simulink model "EZEStEnCtrl"  (R2018b)
settings: Solver=FixedStepDiscrete  StartTime=0.0  StopTime=10.0  FixedStep=0.01  RelTol=1e-3  EnableMultiTasking=on
undefined symbols (not defined in the file or in its folder): data, DrvStFtEn_Clear, DrvStFtEn_Set, KeSMSwSecRwLtStEasyEntryCllsnPt_Val, KeSMSwSecRwRtStEasyEntryCllsnPt_Val, PassStFtEn_Clear, PassStFtEn_Set, SecRwLtStArmScrnEn_Clear, SecRwLtStArmScrnEn_Set, SecRwLtStBkReclnEn_Clear, SecRwLtStBkReclnEn_Set, SecRwLtStFwdBkwdEn_Clear, SecRwLtStFwdBkwdEn_Set, SecRwLtStLgrstUpwdDnwdEn_Clear, SecRwLtStLgrstUpwdDnwdEn_Set, SecRwLtStLtwdRtwdEn_Clear, SecRwLtStLtwdRtwdEn_Set, SecRwRtStArmScrnEn_Clear, SecRwRtStArmScrnEn_Set, SecRwRtStBkReclnEn_Clear, SecRwRtStBkReclnEn_Set, SecRwRtStFwdBkwdEn_Clear, SecRwRtStFwdBkwdEn_Set, SecRwRtStLgrstUpwdDnwdEn_Clear, SecRwRtStLgrstUpwdDnwdEn_Set, SecRwRtStLtwdRtwdEn_Clear, SecRwRtStLtwdRtwdEn_Set, ThdRwLtStBkReclnEn_Clear, ThdRwLtStBkReclnEn_Set, ThdRwLtStCshnFldEn_Clear, ThdRwLtStCshnFldEn_Set, ThdRwLtStFwdBkwdEn_Clear, ThdRwLtStFwdBkwdEn_Set, ThdRwRtStBkReclnEn_Clear, ThdRwRtStBkReclnEn_Set, ThdRwRtStCshnFldEn_Clear, ThdRwRtStCshnFldEn_Set, ThdRwRtStFwdBkwdEn_Clear, ThdRwRtStFwdBkwdEn_Set
libraries: simulink x1
settings Model: Creator=sn2xws  LastModifiedBy=sn2xws
settings DataIOCC: SaveFormat=StructureWithTime
settings OptimizationCC: DefaultParameterBehavior=Inlined  UseFloatMulNetSlope=on  InlineInvariantSignals=on  PassReuseOutputArgsAs=Individual arguments  ZeroExternalMemoryAtStartup=off  ZeroInternalMemoryAtStartup=off  NoFixptDivByZeroProtection=on  EfficientFloat2IntCast=on  LifeSpan=1  OptimizeBlockOrder=speed  DifferentSizesBufferReuse=on
settings DebuggingCC: ParameterTunabilityLossMsg=error
settings HardwareCC: ProdLongLongMode=on
settings ModelReferenceCC: ModelReferenceNumInstancesAllowed=Single
settings SFSimCC: MATLABDynamicMemAlloc=off
settings RTWCC: SystemTargetFile=autosar.tlc  GenCodeOnly=on  TemplateMakefile=ert_default_tmf  Description=AUTOSAR  GenerateReport=on  IncludeHyperlinkInReport=on  LaunchReport=on  GenerateTraceInfo=on  GenerateTraceReport=on  GenerateTraceReportSl=on  GenerateTraceReportSf=on  GenerateTraceReportEml=on  GenerateCodeMetricsReport=on
settings CodeAppCC: ForceParamTrailComments=on  IgnoreCustomStorageClasses=off  OperatorAnnotations=on  SimulinkDataObjDesc=on  SFDataObjDesc=on  CustomSymbolStrGlobalVar=rt$N$M  CustomSymbolStrType=$N$M  CustomSymbolStrFcn=$N$M$F  CustomSymbolStrMacro=$N$M  InsertBlockDesc=on
settings STFCustomTargetCC: TargetLangStandard=C99 (ISO)  MultiwordLength=256  ParMdlRefBuildCompliant=on  CompOptLevelCompliant=on  IncludeMdlTerminateFcn=off  CombineOutputUpdateFcns=on  CombineSignalStateStructs=on  SuppressErrorStatus=on  ERTCustomFileBanners=on  SupportAbsoluteTime=off  SupportNonFinite=off  SupportComplex=off  SupportContinuousTime=off  SupportNonInlinedSFcns=off  RemoveResetFunc=on  MATLABClassNameForMDSCustomization=Simulink.SoftwareTarget.ERTCustomization  AutosarCompliant=on  UseToolchainInfoCompliant=on  LookupTableObjectStructAxisOrder=2,1,3,4,...  LUTObjectStructOrderEvenSpacing=Size,Table,Breakpoints  SystemTargetFile=autosar.tlc
settings ERTTargetCC: TargetLangStandard=C99 (ISO)  ConcurrentExecutionCompliant=off  IncludeMdlTerminateFcn=off  CombineSignalStateStructs=on  SuppressErrorStatus=on  SupportAbsoluteTime=off  SupportNonFinite=off  SupportComplex=off  ModelStepFunctionPrototypeControlCompliant=off  CPPClassGenCompliant=off  AutosarCompliant=on  LookupTableObjectStructAxisOrder=2,1,3,4,...  LUTObjectStructOrderEvenSpacing=Size,Table,Breakpoints  InlinedParameterPlacement=NonHierarchical  ERTCustomFileTemplate=example_file_process.tlc  ERTFilePackagingFormat=CompactWithDataFile

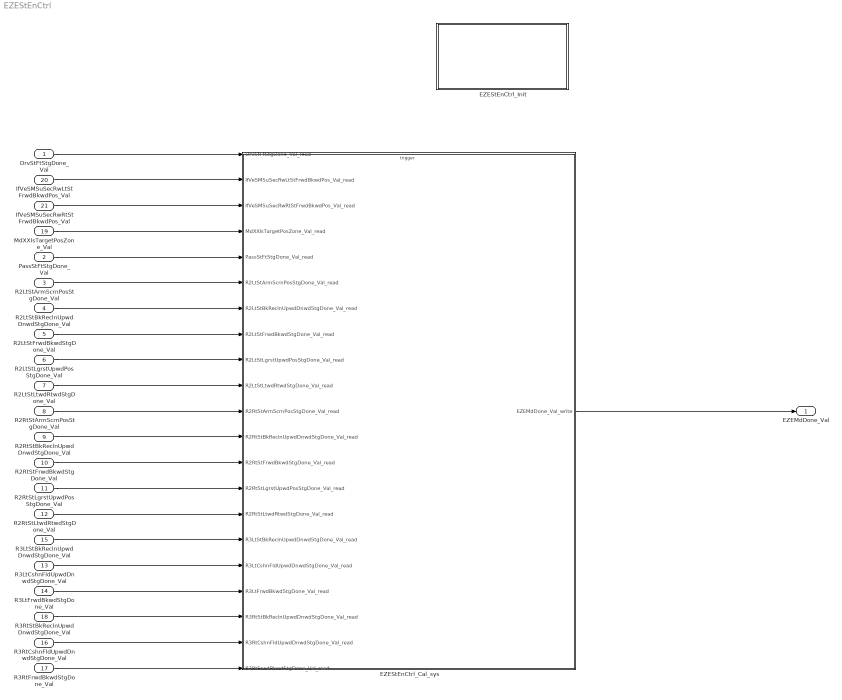
== system EZEStEnCtrl ==
  DrvStFtStgDone_Val : Inport  OutDataTypeStr=boolean  PortDimensions=1
  PassStFtStgDone_Val : Inport  Port=2  OutDataTypeStr=boolean  PortDimensions=1
  R2LtStArmScrnPosStgDone_Val : Inport  Port=3  OutDataTypeStr=boolean  PortDimensions=1
  R2LtStBkReclnUpwdDnwdStgDone_Val : Inport  Port=4  OutDataTypeStr=boolean  PortDimensions=1
  R2LtStFrwdBkwdStgDone_Val : Inport  Port=5  OutDataTypeStr=boolean  PortDimensions=1
  R2LtStLgrstUpwdPosStgDone_Val : Inport  Port=6  OutDataTypeStr=boolean  PortDimensions=1
  R2LtStLtwdRtwdStgDone_Val : Inport  Port=7  OutDataTypeStr=boolean  PortDimensions=1
  R2RtStArmScrnPosStgDone_Val : Inport  Port=8  OutDataTypeStr=boolean  PortDimensions=1
  R2RtStBkReclnUpwdDnwdStgDone_Val : Inport  Port=9  OutDataTypeStr=boolean  PortDimensions=1
  R2RtStFrwdBkwdStgDone_Val : Inport  Port=10  OutDataTypeStr=boolean  PortDimensions=1
  R2RtStLgrstUpwdPosStgDone_Val : Inport  Port=11  OutDataTypeStr=boolean  PortDimensions=1
  R2RtStLtwdRtwdStgDone_Val : Inport  Port=12  OutDataTypeStr=boolean  PortDimensions=1
  R3LtCshnFldUpwdDnwdStgDone_Val : Inport  Port=13  OutDataTypeStr=boolean  PortDimensions=1
  R3LtFrwdBkwdStgDone_Val : Inport  Port=14  OutDataTypeStr=boolean  PortDimensions=1
  R3LtStBkReclnUpwdDnwdStgDone_Val : Inport  Port=15  OutDataTypeStr=boolean  PortDimensions=1
  R3RtCshnFldUpwdDnwdStgDone_Val : Inport  Port=16  OutDataTypeStr=boolean  PortDimensions=1
  R3RtFrwdBkwdStgDone_Val : Inport  Port=17  OutDataTypeStr=boolean  PortDimensions=1
  R3RtStBkReclnUpwdDnwdStgDone_Val : Inport  Port=18  OutDataTypeStr=boolean  PortDimensions=1
  MdXXIsTargetPosZone_Val : Inport  Port=19  OutDataTypeStr=uint32  PortDimensions=1
  IfVeSMSuSecRwLtStFrwdBkwdPos_Val : Inport  Port=20  OutDataTypeStr=uint16  PortDimensions=1
  IfVeSMSuSecRwRtStFrwdBkwdPos_Val : Inport  Port=21  OutDataTypeStr=uint16  PortDimensions=1
  EZEStEnCtrl_Cal_sys : Subsystem
  EZEStEnCtrl_Init : Subsystem
  EZEMdDone_Val : Outport  OutDataTypeStr=uint8  PortDimensions=1
  wires:
  DrvStFtStgDone_Val/1 -> EZEStEnCtrl_Cal_sys/1(DrvStFtStgDone_Val_read)
  PassStFtStgDone_Val/1 -> EZEStEnCtrl_Cal_sys/5(PassStFtStgDone_Val_read)
  R2LtStArmScrnPosStgDone_Val/1 -> EZEStEnCtrl_Cal_sys/6(R2LtStArmScrnPosStgDone_Val_read)
  R2LtStBkReclnUpwdDnwdStgDone_Val/1 -> EZEStEnCtrl_Cal_sys/7(R2LtStBkReclnUpwdDnwdStgDone_Val_read)
  R2LtStFrwdBkwdStgDone_Val/1 -> EZEStEnCtrl_Cal_sys/8(R2LtStFrwdBkwdStgDone_Val_read)
  R2LtStLgrstUpwdPosStgDone_Val/1 -> EZEStEnCtrl_Cal_sys/9(R2LtStLgrstUpwdPosStgDone_Val_read)
  R2LtStLtwdRtwdStgDone_Val/1 -> EZEStEnCtrl_Cal_sys/10(R2LtStLtwdRtwdStgDone_Val_read)
  R2RtStArmScrnPosStgDone_Val/1 -> EZEStEnCtrl_Cal_sys/11(R2RtStArmScrnPosStgDone_Val_read)
  R2RtStBkReclnUpwdDnwdStgDone_Val/1 -> EZEStEnCtrl_Cal_sys/12(R2RtStBkReclnUpwdDnwdStgDone_Val_read)
  R2RtStFrwdBkwdStgDone_Val/1 -> EZEStEnCtrl_Cal_sys/13(R2RtStFrwdBkwdStgDone_Val_read)
  R2RtStLgrstUpwdPosStgDone_Val/1 -> EZEStEnCtrl_Cal_sys/14(R2RtStLgrstUpwdPosStgDone_Val_read)
  R2RtStLtwdRtwdStgDone_Val/1 -> EZEStEnCtrl_Cal_sys/15(R2RtStLtwdRtwdStgDone_Val_read)
  R3LtCshnFldUpwdDnwdStgDone_Val/1 -> EZEStEnCtrl_Cal_sys/17(R3LtCshnFldUpwdDnwdStgDone_Val_read)
  R3LtFrwdBkwdStgDone_Val/1 -> EZEStEnCtrl_Cal_sys/18(R3LtFrwdBkwdStgDone_Val_read)
  R3LtStBkReclnUpwdDnwdStgDone_Val/1 -> EZEStEnCtrl_Cal_sys/16(R3LtStBkReclnUpwdDnwdStgDone_Val_read)
  R3RtCshnFldUpwdDnwdStgDone_Val/1 -> EZEStEnCtrl_Cal_sys/20(R3RtCshnFldUpwdDnwdStgDone_Val_read)
  R3RtFrwdBkwdStgDone_Val/1 -> EZEStEnCtrl_Cal_sys/21(R3RtFrwdBkwdStgDone_Val_read)
  R3RtStBkReclnUpwdDnwdStgDone_Val/1 -> EZEStEnCtrl_Cal_sys/19(R3RtStBkReclnUpwdDnwdStgDone_Val_read)
  MdXXIsTargetPosZone_Val/1 -> EZEStEnCtrl_Cal_sys/4(MdXXIsTargetPosZone_Val_read)
  EZEStEnCtrl_Cal_sys/1(EZEMdDone_Val_write) -> EZEMdDone_Val/1
  IfVeSMSuSecRwLtStFrwdBkwdPos_Val/1 -> EZEStEnCtrl_Cal_sys/2(IfVeSMSuSecRwLtStFrwdBkwdPos_Val_read)
  IfVeSMSuSecRwRtStFrwdBkwdPos_Val/1 -> EZEStEnCtrl_Cal_sys/3(IfVeSMSuSecRwRtStFrwdBkwdPos_Val_read)

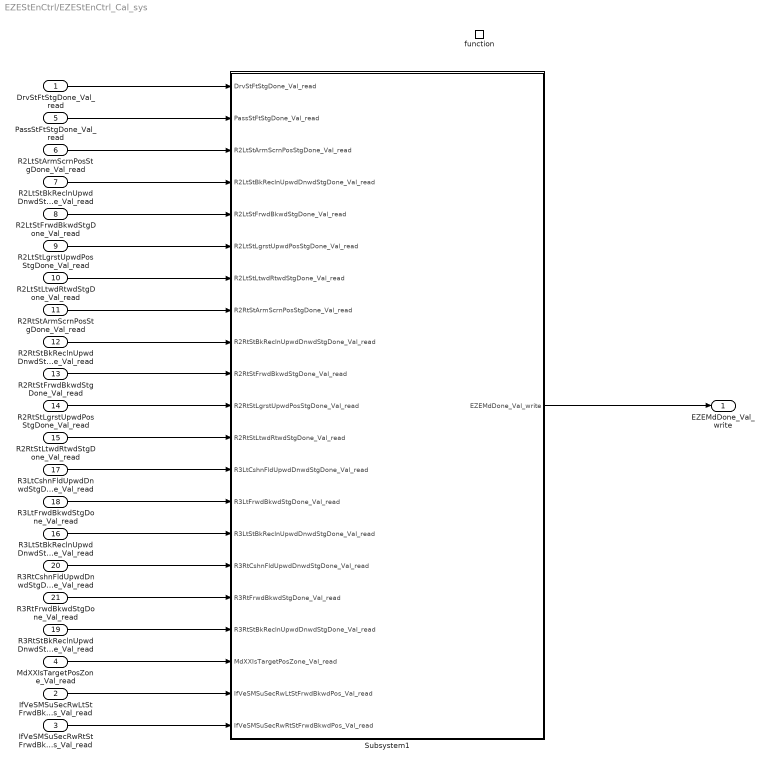
== system EZEStEnCtrl/EZEStEnCtrl_Cal_sys ==
  DrvStFtStgDone_Val_read : Inport
  IfVeSMSuSecRwLtStFrwdBkwdPos_Val_read : Inport  Port=2
  IfVeSMSuSecRwRtStFrwdBkwdPos_Val_read : Inport  Port=3
  MdXXIsTargetPosZone_Val_read : Inport  Port=4
  PassStFtStgDone_Val_read : Inport  Port=5
  R2LtStArmScrnPosStgDone_Val_read : Inport  Port=6
  R2LtStBkReclnUpwdDnwdStgDone_Val_read : Inport  Port=7
  R2LtStFrwdBkwdStgDone_Val_read : Inport  Port=8
  R2LtStLgrstUpwdPosStgDone_Val_read : Inport  Port=9
  R2LtStLtwdRtwdStgDone_Val_read : Inport  Port=10
  R2RtStArmScrnPosStgDone_Val_read : Inport  Port=11
  R2RtStBkReclnUpwdDnwdStgDone_Val_read : Inport  Port=12
  R2RtStFrwdBkwdStgDone_Val_read : Inport  Port=13
  R2RtStLgrstUpwdPosStgDone_Val_read : Inport  Port=14
  R2RtStLtwdRtwdStgDone_Val_read : Inport  Port=15
  R3LtStBkReclnUpwdDnwdStgDone_Val_read : Inport  Port=16
  R3LtCshnFldUpwdDnwdStgDone_Val_read : Inport  Port=17
  R3LtFrwdBkwdStgDone_Val_read : Inport  Port=18
  R3RtStBkReclnUpwdDnwdStgDone_Val_read : Inport  Port=19
  R3RtCshnFldUpwdDnwdStgDone_Val_read : Inport  Port=20
  R3RtFrwdBkwdStgDone_Val_read : Inport  Port=21
  function : TriggerPort  TriggerType=function-call  IsSimulinkFunction=on  FunctionName=EZEStEnCtrl_Cal  VariantControl=(inherit)
  Subsystem1 : Subsystem
  EZEMdDone_Val_write : Outport
      settings: EnsureOutportIsVirtual=on
  wires:
  Subsystem1/1(EZEMdDone_Val_write) -> EZEMdDone_Val_write/1
  DrvStFtStgDone_Val_read/1 -> Subsystem1/1(DrvStFtStgDone_Val_read)
  PassStFtStgDone_Val_read/1 -> Subsystem1/2(PassStFtStgDone_Val_read)
  R2LtStArmScrnPosStgDone_Val_read/1 -> Subsystem1/3(R2LtStArmScrnPosStgDone_Val_read)
  R2LtStBkReclnUpwdDnwdStgDone_Val_read/1 -> Subsystem1/4(R2LtStBkReclnUpwdDnwdStgDone_Val_read)
  R2LtStFrwdBkwdStgDone_Val_read/1 -> Subsystem1/5(R2LtStFrwdBkwdStgDone_Val_read)
  R2LtStLgrstUpwdPosStgDone_Val_read/1 -> Subsystem1/6(R2LtStLgrstUpwdPosStgDone_Val_read)
  R2LtStLtwdRtwdStgDone_Val_read/1 -> Subsystem1/7(R2LtStLtwdRtwdStgDone_Val_read)
  R2RtStLgrstUpwdPosStgDone_Val_read/1 -> Subsystem1/11(R2RtStLgrstUpwdPosStgDone_Val_read)
  R2RtStLtwdRtwdStgDone_Val_read/1 -> Subsystem1/12(R2RtStLtwdRtwdStgDone_Val_read)
  R2RtStArmScrnPosStgDone_Val_read/1 -> Subsystem1/8(R2RtStArmScrnPosStgDone_Val_read)
  R2RtStBkReclnUpwdDnwdStgDone_Val_read/1 -> Subsystem1/9(R2RtStBkReclnUpwdDnwdStgDone_Val_read)
  R2RtStFrwdBkwdStgDone_Val_read/1 -> Subsystem1/10(R2RtStFrwdBkwdStgDone_Val_read)
  R3LtCshnFldUpwdDnwdStgDone_Val_read/1 -> Subsystem1/13(R3LtCshnFldUpwdDnwdStgDone_Val_read)
  R3LtFrwdBkwdStgDone_Val_read/1 -> Subsystem1/14(R3LtFrwdBkwdStgDone_Val_read)
  R3LtStBkReclnUpwdDnwdStgDone_Val_read/1 -> Subsystem1/15(R3LtStBkReclnUpwdDnwdStgDone_Val_read)
  R3RtCshnFldUpwdDnwdStgDone_Val_read/1 -> Subsystem1/16(R3RtCshnFldUpwdDnwdStgDone_Val_read)
  R3RtFrwdBkwdStgDone_Val_read/1 -> Subsystem1/17(R3RtFrwdBkwdStgDone_Val_read)
  R3RtStBkReclnUpwdDnwdStgDone_Val_read/1 -> Subsystem1/18(R3RtStBkReclnUpwdDnwdStgDone_Val_read)
  MdXXIsTargetPosZone_Val_read/1 -> Subsystem1/19(MdXXIsTargetPosZone_Val_read)
  IfVeSMSuSecRwLtStFrwdBkwdPos_Val_read/1 -> Subsystem1/20(IfVeSMSuSecRwLtStFrwdBkwdPos_Val_read)
  IfVeSMSuSecRwRtStFrwdBkwdPos_Val_read/1 -> Subsystem1/21(IfVeSMSuSecRwRtStFrwdBkwdPos_Val_read)

== system EZEStEnCtrl/EZEStEnCtrl_Init ==
  Event Listener : EventListener  EventName=reset

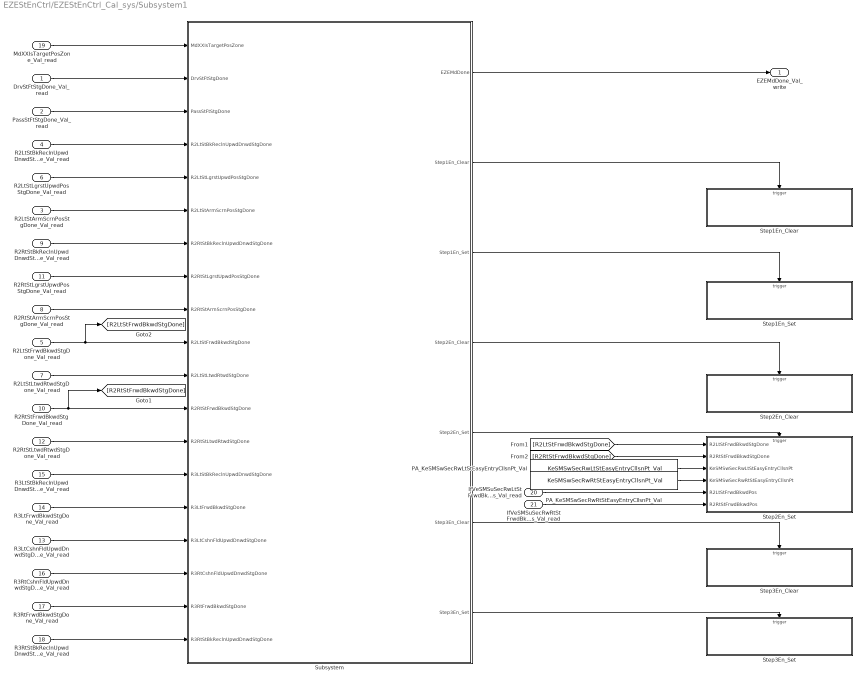
== system EZEStEnCtrl/EZEStEnCtrl_Cal_sys/Subsystem1 ==
  DrvStFtStgDone_Val_read : Inport
  PassStFtStgDone_Val_read : Inport  Port=2
  R2LtStArmScrnPosStgDone_Val_read : Inport  Port=3
  R2LtStBkReclnUpwdDnwdStgDone_Val_read : Inport  Port=4
  R2LtStFrwdBkwdStgDone_Val_read : Inport  Port=5
  R2LtStLgrstUpwdPosStgDone_Val_read : Inport  Port=6
  R2LtStLtwdRtwdStgDone_Val_read : Inport  Port=7
  R2RtStArmScrnPosStgDone_Val_read : Inport  Port=8
  R2RtStBkReclnUpwdDnwdStgDone_Val_read : Inport  Port=9
  R2RtStFrwdBkwdStgDone_Val_read : Inport  Port=10
  R2RtStLgrstUpwdPosStgDone_Val_read : Inport  Port=11
  R2RtStLtwdRtwdStgDone_Val_read : Inport  Port=12
  R3LtCshnFldUpwdDnwdStgDone_Val_read : Inport  Port=13
  R3LtFrwdBkwdStgDone_Val_read : Inport  Port=14
  R3LtStBkReclnUpwdDnwdStgDone_Val_read : Inport  Port=15
  R3RtCshnFldUpwdDnwdStgDone_Val_read : Inport  Port=16
  R3RtFrwdBkwdStgDone_Val_read : Inport  Port=17
  R3RtStBkReclnUpwdDnwdStgDone_Val_read : Inport  Port=18
  MdXXIsTargetPosZone_Val_read : Inport  Port=19
  IfVeSMSuSecRwLtStFrwdBkwdPos_Val_read : Inport  Port=20
  IfVeSMSuSecRwRtStFrwdBkwdPos_Val_read : Inport  Port=21
  PA_KeSMSwSecRwLtStEasyEntryCllsnPt_Val : Constant  Value=KeSMSwSecRwLtStEasyEntryCllsnPt_Val
  PA_KeSMSwSecRwRtStEasyEntryCllsnPt_Val : Constant  Value=KeSMSwSecRwRtStEasyEntryCllsnPt_Val
  Step1En_Clear : Subsystem
  Step1En_Set : Subsystem
  Step2En_Clear : Subsystem
  Step2En_Set : Subsystem
  Step3En_Clear : Subsystem
  Step3En_Set : Subsystem
  Subsystem : Subsystem
  EZEMdDone_Val_write : Outport
      settings: EnsureOutportIsVirtual=on
  wires:
  Subsystem/3(Step1En_Set) -> Step1En_Set/Trigger
  R2LtStFrwdBkwdStgDone_Val_read/1 -> [R2LtStFrwdBkwdStgDone], Subsystem/10(R2LtStFrwdBkwdStgDone)
  R2RtStLgrstUpwdPosStgDone_Val_read/1 -> Subsystem/8(R2RtStLgrstUpwdPosStgDone)
  [R2LtStFrwdBkwdStgDone] -> Step2En_Set/1(R2LtStFrwdBkwdStgDone)
  Subsystem/5(Step2En_Set) -> Step2En_Set/Trigger
  R2LtStLtwdRtwdStgDone_Val_read/1 -> Subsystem/11(R2LtStLtwdRtwdStgDone)
  DrvStFtStgDone_Val_read/1 -> Subsystem/2(DrvStFtStgDone)
  R3LtFrwdBkwdStgDone_Val_read/1 -> Subsystem/15(R3LtFrwdBkwdStgDone)
  PA_KeSMSwSecRwLtStEasyEntryCllsnPt_Val/1 -> Step2En_Set/3(KeSMSwSecRwLtStEasyEntryCllsnPt)
  R2RtStFrwdBkwdStgDone_Val_read/1 -> [R2RtStFrwdBkwdStgDone], Subsystem/12(R2RtStFrwdBkwdStgDone)
  R3RtFrwdBkwdStgDone_Val_read/1 -> Subsystem/18(R3RtFrwdBkwdStgDone)
  Subsystem/1(EZEMdDone) -> EZEMdDone_Val_write/1
  R3LtStBkReclnUpwdDnwdStgDone_Val_read/1 -> Subsystem/14(R3LtStBkReclnUpwdDnwdStgDone)
  [R2RtStFrwdBkwdStgDone] -> Step2En_Set/2(R2RtStFrwdBkwdStgDone)
  Subsystem/7(Step3En_Set) -> Step3En_Set/Trigger
  R2RtStLtwdRtwdStgDone_Val_read/1 -> Subsystem/13(R2RtStLtwdRtwdStgDone)
  R3LtCshnFldUpwdDnwdStgDone_Val_read/1 -> Subsystem/16(R3LtCshnFldUpwdDnwdStgDone)
  MdXXIsTargetPosZone_Val_read/1 -> Subsystem/1(MdXXIsTargetPosZone)
  R2RtStArmScrnPosStgDone_Val_read/1 -> Subsystem/9(R2RtStArmScrnPosStgDone)
  R2RtStBkReclnUpwdDnwdStgDone_Val_read/1 -> Subsystem/7(R2RtStBkReclnUpwdDnwdStgDone)
  PassStFtStgDone_Val_read/1 -> Subsystem/3(PassStFtStgDone)
  R2LtStArmScrnPosStgDone_Val_read/1 -> Subsystem/6(R2LtStArmScrnPosStgDone)
  Subsystem/6(Step3En_Clear) -> Step3En_Clear/Trigger
  R2LtStBkReclnUpwdDnwdStgDone_Val_read/1 -> Subsystem/4(R2LtStBkReclnUpwdDnwdStgDone)
  R3RtStBkReclnUpwdDnwdStgDone_Val_read/1 -> Subsystem/19(R3RtStBkReclnUpwdDnwdStgDone)
  Subsystem/4(Step2En_Clear) -> Step2En_Clear/Trigger
  PA_KeSMSwSecRwRtStEasyEntryCllsnPt_Val/1 -> Step2En_Set/4(KeSMSwSecRwRtStEasyEntryCllsnPt)
  Subsystem/2(Step1En_Clear) -> Step1En_Clear/Trigger
  R3RtCshnFldUpwdDnwdStgDone_Val_read/1 -> Subsystem/17(R3RtCshnFldUpwdDnwdStgDone)
  IfVeSMSuSecRwLtStFrwdBkwdPos_Val_read/1 -> Step2En_Set/5(R2LtStFrwdBkwdPos)
  IfVeSMSuSecRwRtStFrwdBkwdPos_Val_read/1 -> Step2En_Set/6(R2RtStFrwdBkwdPos)
  R2LtStLgrstUpwdPosStgDone_Val_read/1 -> Subsystem/5(R2LtStLgrstUpwdPosStgDone)

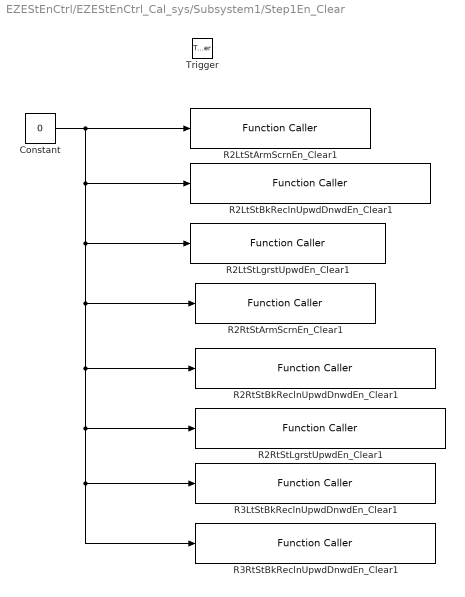
== system EZEStEnCtrl/EZEStEnCtrl_Cal_sys/Subsystem1/Step1En_Clear ==
  Trigger : TriggerPort  TriggerType=function-call  VariantControl=Variant  PortDimensions=1
  Constant : Constant  Value=0  OutDataTypeStr=uint8
  R2LtStArmScrnEn_Clear1 : FunctionCaller  FunctionPrototype=SecRwLtStArmScrnEn_Clear(data)  InputArgumentSpecifications=uint8(1)
  R2LtStBkReclnUpwdDnwdEn_Clear1 : FunctionCaller  FunctionPrototype=SecRwLtStBkReclnEn_Clear(data)  InputArgumentSpecifications=uint8(1)
  R2LtStLgrstUpwdEn_Clear1 : FunctionCaller  FunctionPrototype=SecRwLtStLgrstUpwdDnwdEn_Clear(data)  InputArgumentSpecifications=uint8(1)
  R2RtStArmScrnEn_Clear1 : FunctionCaller  FunctionPrototype=SecRwRtStArmScrnEn_Clear(data)  InputArgumentSpecifications=uint8(1)
  R2RtStBkReclnUpwdDnwdEn_Clear1 : FunctionCaller  FunctionPrototype=SecRwRtStBkReclnEn_Clear(data)  InputArgumentSpecifications=uint8(1)
  R2RtStLgrstUpwdEn_Clear1 : FunctionCaller  FunctionPrototype=SecRwRtStLgrstUpwdDnwdEn_Clear(data)  InputArgumentSpecifications=uint8(1)
  R3LtStBkReclnUpwdDnwdEn_Clear1 : FunctionCaller  FunctionPrototype=ThdRwLtStBkReclnEn_Clear(data)  InputArgumentSpecifications=uint8(1)
  R3RtStBkReclnUpwdDnwdEn_Clear1 : FunctionCaller  FunctionPrototype=ThdRwRtStBkReclnEn_Clear(data)  InputArgumentSpecifications=uint8(1)
  wires:
  Constant/1 -> R3RtStBkReclnUpwdDnwdEn_Clear1/1, R3LtStBkReclnUpwdDnwdEn_Clear1/1, R2RtStLgrstUpwdEn_Clear1/1, R2RtStBkReclnUpwdDnwdEn_Clear1/1, R2RtStArmScrnEn_Clear1/1, R2LtStLgrstUpwdEn_Clear1/1, R2LtStBkReclnUpwdDnwdEn_Clear1/1, R2LtStArmScrnEn_Clear1/1

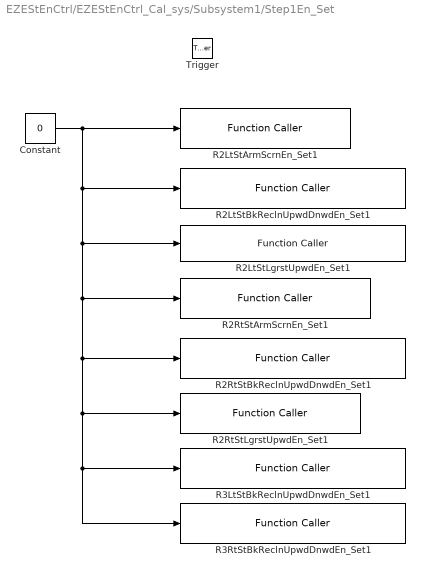
== system EZEStEnCtrl/EZEStEnCtrl_Cal_sys/Subsystem1/Step1En_Set ==
  Trigger : TriggerPort  TriggerType=function-call  VariantControl=Variant  PortDimensions=1
  Constant : Constant  Value=0  OutDataTypeStr=uint8
  R2LtStArmScrnEn_Set1 : FunctionCaller  FunctionPrototype=SecRwLtStArmScrnEn_Set(data)  InputArgumentSpecifications=uint8(1)
  R2LtStBkReclnUpwdDnwdEn_Set1 : FunctionCaller  FunctionPrototype=SecRwLtStBkReclnEn_Set(data)  InputArgumentSpecifications=uint8(1)
  R2LtStLgrstUpwdEn_Set1 : FunctionCaller  FunctionPrototype=SecRwLtStLgrstUpwdDnwdEn_Set(data)  InputArgumentSpecifications=uint8(1)
  R2RtStArmScrnEn_Set1 : FunctionCaller  FunctionPrototype=SecRwRtStArmScrnEn_Set(data)  InputArgumentSpecifications=uint8(1)
  R2RtStBkReclnUpwdDnwdEn_Set1 : FunctionCaller  FunctionPrototype=SecRwRtStBkReclnEn_Set(data)  InputArgumentSpecifications=uint8(1)
  R2RtStLgrstUpwdEn_Set1 : FunctionCaller  FunctionPrototype=SecRwRtStLgrstUpwdDnwdEn_Set(data)  InputArgumentSpecifications=uint8(1)
  R3LtStBkReclnUpwdDnwdEn_Set1 : FunctionCaller  FunctionPrototype=ThdRwLtStBkReclnEn_Set(data)  InputArgumentSpecifications=uint8(1)
  R3RtStBkReclnUpwdDnwdEn_Set1 : FunctionCaller  FunctionPrototype=ThdRwRtStBkReclnEn_Set(data)  InputArgumentSpecifications=uint8(1)
  wires:
  Constant/1 -> R2LtStLgrstUpwdEn_Set1/1, R2RtStArmScrnEn_Set1/1, R2RtStLgrstUpwdEn_Set1/1, R3RtStBkReclnUpwdDnwdEn_Set1/1, R3LtStBkReclnUpwdDnwdEn_Set1/1, R2RtStBkReclnUpwdDnwdEn_Set1/1, R2LtStBkReclnUpwdDnwdEn_Set1/1, R2LtStArmScrnEn_Set1/1

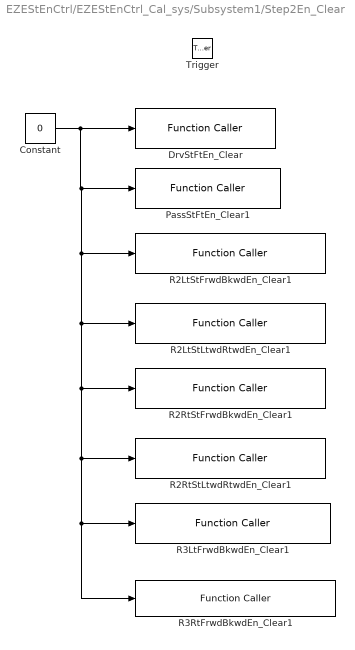
== system EZEStEnCtrl/EZEStEnCtrl_Cal_sys/Subsystem1/Step2En_Clear ==
  Trigger : TriggerPort  TriggerType=function-call  VariantControl=Variant  PortDimensions=1
  Constant : Constant  Value=0  OutDataTypeStr=uint8
  DrvStFtEn_Clear : FunctionCaller  FunctionPrototype=DrvStFtEn_Clear(data)  InputArgumentSpecifications=uint8(1)
  PassStFtEn_Clear1 : FunctionCaller  FunctionPrototype=PassStFtEn_Clear(data)  InputArgumentSpecifications=uint8(1)
  R2LtStFrwdBkwdEn_Clear1 : FunctionCaller  FunctionPrototype=SecRwLtStFwdBkwdEn_Clear(data)  InputArgumentSpecifications=uint8(1)
  R2LtStLtwdRtwdEn_Clear1 : FunctionCaller  FunctionPrototype=SecRwLtStLtwdRtwdEn_Clear(data)  InputArgumentSpecifications=uint8(1)
  R2RtStFrwdBkwdEn_Clear1 : FunctionCaller  FunctionPrototype=SecRwRtStFwdBkwdEn_Clear(data)  InputArgumentSpecifications=uint8(1)
  R2RtStLtwdRtwdEn_Clear1 : FunctionCaller  FunctionPrototype=SecRwRtStLtwdRtwdEn_Clear(data)  InputArgumentSpecifications=uint8(1)
  R3LtFrwdBkwdEn_Clear1 : FunctionCaller  FunctionPrototype=ThdRwLtStFwdBkwdEn_Clear(data)  InputArgumentSpecifications=uint8(1)
  R3RtFrwdBkwdEn_Clear1 : FunctionCaller  FunctionPrototype=ThdRwRtStFwdBkwdEn_Clear(data)  InputArgumentSpecifications=uint8(1)
  wires:
  Constant/1 -> R2RtStFrwdBkwdEn_Clear1/1, R2RtStLtwdRtwdEn_Clear1/1, R3RtFrwdBkwdEn_Clear1/1, R3LtFrwdBkwdEn_Clear1/1, R2LtStLtwdRtwdEn_Clear1/1, R2LtStFrwdBkwdEn_Clear1/1, PassStFtEn_Clear1/1, DrvStFtEn_Clear/1

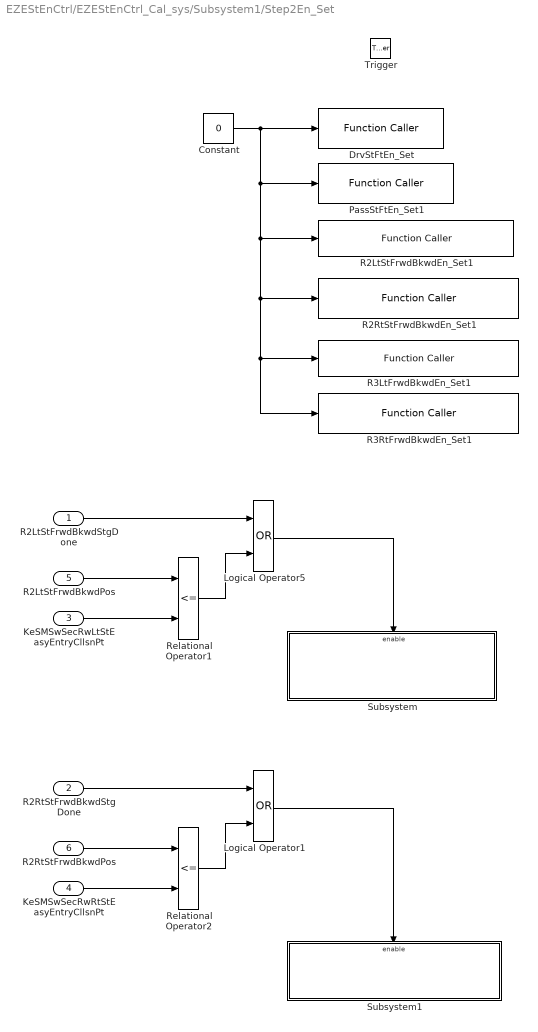
== system EZEStEnCtrl/EZEStEnCtrl_Cal_sys/Subsystem1/Step2En_Set ==
  R2LtStFrwdBkwdStgDone : Inport
  R2RtStFrwdBkwdStgDone : Inport  Port=2
  KeSMSwSecRwLtStEasyEntryCllsnPt : Inport  Port=3
  KeSMSwSecRwRtStEasyEntryCllsnPt : Inport  Port=4
  R2LtStFrwdBkwdPos : Inport  Port=5
  R2RtStFrwdBkwdPos : Inport  Port=6
  Trigger : TriggerPort  TriggerType=function-call  VariantControl=Variant  PortDimensions=1
  Constant : Constant  Value=0  OutDataTypeStr=uint8
  DrvStFtEn_Set : FunctionCaller  FunctionPrototype=DrvStFtEn_Set(data)  InputArgumentSpecifications=uint8(1)
  Logical Operator1 : Logic  Operator=OR  AllPortsSameDT=off  OutDataTypeStr=boolean
  Logical Operator5 : Logic  Operator=OR  AllPortsSameDT=off  OutDataTypeStr=boolean
  PassStFtEn_Set1 : FunctionCaller  FunctionPrototype=PassStFtEn_Set(data)  InputArgumentSpecifications=uint8(1)
  R2LtStFrwdBkwdEn_Set1 : FunctionCaller  FunctionPrototype=SecRwLtStFwdBkwdEn_Set(data)  InputArgumentSpecifications=uint8(1)
  R2RtStFrwdBkwdEn_Set1 : FunctionCaller  FunctionPrototype=SecRwRtStFwdBkwdEn_Set(data)  InputArgumentSpecifications=uint8(1)
  R3LtFrwdBkwdEn_Set1 : FunctionCaller  FunctionPrototype=ThdRwLtStFwdBkwdEn_Set(data)  InputArgumentSpecifications=uint8(1)
  R3RtFrwdBkwdEn_Set1 : FunctionCaller  FunctionPrototype=ThdRwRtStFwdBkwdEn_Set(data)  InputArgumentSpecifications=uint8(1)
  Relational Operator1 : RelationalOperator  Operator=<=  OutDataTypeStr=boolean  RndMeth=Simplest
  Relational Operator2 : RelationalOperator  Operator=<=  OutDataTypeStr=boolean  RndMeth=Simplest
  Subsystem : Subsystem
  Subsystem1 : Subsystem
  wires:
  Constant/1 -> PassStFtEn_Set1/1, R2LtStFrwdBkwdEn_Set1/1, R3RtFrwdBkwdEn_Set1/1, R3LtFrwdBkwdEn_Set1/1, R2RtStFrwdBkwdEn_Set1/1, DrvStFtEn_Set/1
  R2LtStFrwdBkwdStgDone/1 -> Logical Operator5/1
  R2LtStFrwdBkwdPos/1 -> Relational Operator1/1
  KeSMSwSecRwLtStEasyEntryCllsnPt/1 -> Relational Operator1/2
  Relational Operator1/1 -> Logical Operator5/2
  Logical Operator5/1 -> Subsystem/Enable
  R2RtStFrwdBkwdStgDone/1 -> Logical Operator1/1
  Relational Operator2/1 -> Logical Operator1/2
  R2RtStFrwdBkwdPos/1 -> Relational Operator2/1
  KeSMSwSecRwRtStEasyEntryCllsnPt/1 -> Relational Operator2/2
  Logical Operator1/1 -> Subsystem1/Enable

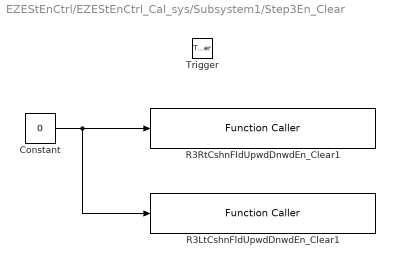
== system EZEStEnCtrl/EZEStEnCtrl_Cal_sys/Subsystem1/Step3En_Clear ==
  Trigger : TriggerPort  TriggerType=function-call  VariantControl=Variant  PortDimensions=1
  Constant : Constant  Value=0  OutDataTypeStr=uint8
  R3LtCshnFldUpwdDnwdEn_Clear1 : FunctionCaller  FunctionPrototype=ThdRwLtStCshnFldEn_Clear(data)  InputArgumentSpecifications=uint8(1)
  R3RtCshnFldUpwdDnwdEn_Clear1 : FunctionCaller  FunctionPrototype=ThdRwRtStCshnFldEn_Clear(data)  InputArgumentSpecifications=uint8(1)
  wires:
  Constant/1 -> R3LtCshnFldUpwdDnwdEn_Clear1/1, R3RtCshnFldUpwdDnwdEn_Clear1/1

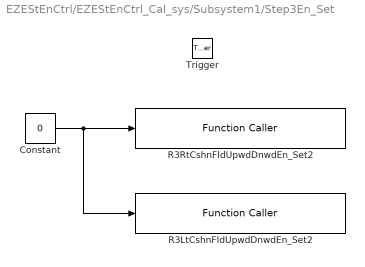
== system EZEStEnCtrl/EZEStEnCtrl_Cal_sys/Subsystem1/Step3En_Set ==
  Trigger : TriggerPort  TriggerType=function-call  VariantControl=Variant  PortDimensions=1
  Constant : Constant  Value=0  OutDataTypeStr=uint8
  R3LtCshnFldUpwdDnwdEn_Set2 : FunctionCaller  FunctionPrototype=ThdRwLtStCshnFldEn_Set(data)  InputArgumentSpecifications=uint8(1)
  R3RtCshnFldUpwdDnwdEn_Set2 : FunctionCaller  FunctionPrototype=ThdRwRtStCshnFldEn_Set(data)  InputArgumentSpecifications=uint8(1)
  wires:
  Constant/1 -> R3LtCshnFldUpwdDnwdEn_Set2/1, R3RtCshnFldUpwdDnwdEn_Set2/1

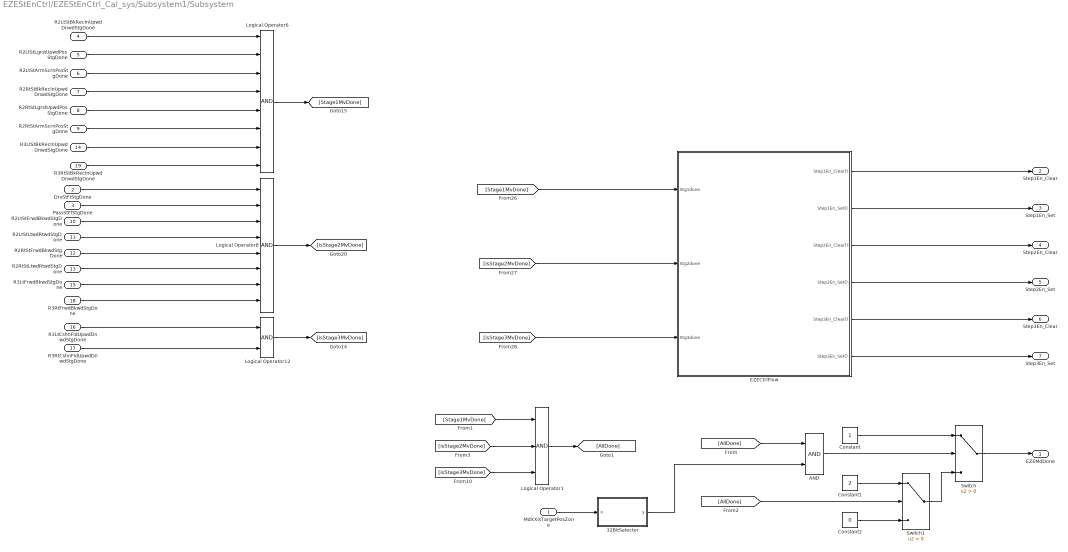
== system EZEStEnCtrl/EZEStEnCtrl_Cal_sys/Subsystem1/Subsystem ==
  MdXXIsTargetPosZone : Inport
  DrvStFtStgDone : Inport  Port=2
  PassStFtStgDone : Inport  Port=3
  R2LtStBkReclnUpwdDnwdStgDone : Inport  Port=4
  R2LtStLgrstUpwdPosStgDone : Inport  Port=5
  R2LtStArmScrnPosStgDone : Inport  Port=6
  R2RtStBkReclnUpwdDnwdStgDone : Inport  Port=7
  R2RtStLgrstUpwdPosStgDone : Inport  Port=8
  R2RtStArmScrnPosStgDone : Inport  Port=9
  R2LtStFrwdBkwdStgDone : Inport  Port=10
  R2LtStLtwdRtwdStgDone : Inport  Port=11
  R2RtStFrwdBkwdStgDone : Inport  Port=12
  R2RtStLtwdRtwdStgDone : Inport  Port=13
  R3LtStBkReclnUpwdDnwdStgDone : Inport  Port=14
  R3LtFrwdBkwdStgDone : Inport  Port=15
  R3LtCshnFldUpwdDnwdStgDone : Inport  Port=16
  R3RtCshnFldUpwdDnwdStgDone : Inport  Port=17
  R3RtFrwdBkwdStgDone : Inport  Port=18
  R3RtStBkReclnUpwdDnwdStgDone : Inport  Port=19
  32BitSelector : Subsystem  mask(32 Bit Selector){BitNum=0}
      mask prompts: BitNum "Select Bit Number"
      mask help: Allows selection of a particular bit (0-31) out of a packed word up to 32 bits long. Output will be true if the bit number selected via the mask parameter is equal to one.
      mask TypeOptions BitNum: 0 | 1 | 2 | 3 | 4 | 5 | 6 | 7 | 8 | 9 | 10 | 11 | 12 | 13 | 14 | 15 | 16 | 17 | 18 | 19 | 20 | 21 | 22 | 23 | 24 | 25 | 26 | 27 | 28 | 29 | 30 | 31
      mask Display:
      | text(0.5, 0.8,'BIT','horizontalAlignment','center')
      | text(0.5, 0.5,'SELECTOR','horizontalAlignment','center')
      | text(0.5, 0.2,['-- Bit ',char(get_param(gcb,'BitNum')),' --'],'horizontalAlignment','center')
  AND : Logic  AllPortsSameDT=off  OutDataTypeStr=boolean
  Constant : Constant  OutDataTypeStr=uint8
  Constant1 : Constant  Value=2  OutDataTypeStr=uint8
  Constant2 : Constant  Value=0  OutDataTypeStr=uint8
  EZECtrlFlow : Stateflow chart  TreatAsAtomicUnit=on
  Logical Operator1 : Logic  Inputs=3  AllPortsSameDT=off  OutDataTypeStr=boolean
  Logical Operator12 : Logic  AllPortsSameDT=off  OutDataTypeStr=boolean
  Logical Operator6 : Logic  Inputs=8  AllPortsSameDT=off  OutDataTypeStr=boolean
  Logical Operator8 : Logic  Inputs=8  AllPortsSameDT=off  OutDataTypeStr=boolean
  Switch : Switch  Criteria=u2 > Threshold
  Switch1 : Switch  Criteria=u2 > Threshold
  EZEMdDone : Outport
  Step1En_Clear : Outport  Port=2
  Step1En_Set : Outport  Port=3
  Step2En_Clear : Outport  Port=4
  Step2En_Set : Outport  Port=5
  Step3En_Clear : Outport  Port=6
  Step3En_Set : Outport  Port=7
  wires:
  R2RtStLtwdRtwdStgDone/1 -> Logical Operator8/6
  PassStFtStgDone/1 -> Logical Operator8/2
  R3RtCshnFldUpwdDnwdStgDone/1 -> Logical Operator12/2
  R2LtStBkReclnUpwdDnwdStgDone/1 -> Logical Operator6/1
  R3LtCshnFldUpwdDnwdStgDone/1 -> Logical Operator12/1
  MdXXIsTargetPosZone/1 -> 32BitSelector/1(x)
  [isStage2MvDone] -> EZECtrlFlow/2(Stg2done)
  [isStage3MvDone] -> EZECtrlFlow/3(Stg3done)
  R2LtStArmScrnPosStgDone/1 -> Logical Operator6/3
  R2LtStFrwdBkwdStgDone/1 -> Logical Operator8/3
  Logical Operator8/1 -> [isStage2MvDone]
  R3LtFrwdBkwdStgDone/1 -> Logical Operator8/7
  Logical Operator12/1 -> [isStage3MvDone]
  R3RtFrwdBkwdStgDone/1 -> Logical Operator8/8
  [isStage2MvDone] -> Logical Operator1/2
  R2LtStLtwdRtwdStgDone/1 -> Logical Operator8/4
  R2LtStLgrstUpwdPosStgDone/1 -> Logical Operator6/2
  [Stage1MvDone] -> Logical Operator1/1
  R3LtStBkReclnUpwdDnwdStgDone/1 -> Logical Operator6/7
  [isStage3MvDone] -> Logical Operator1/3
  R2RtStFrwdBkwdStgDone/1 -> Logical Operator8/5
  R2RtStArmScrnPosStgDone/1 -> Logical Operator6/6
  R2RtStLgrstUpwdPosStgDone/1 -> Logical Operator6/5
  Logical Operator6/1 -> [Stage1MvDone]
  Logical Operator1/1 -> [AllDone]
  DrvStFtStgDone/1 -> Logical Operator8/1
  R2RtStBkReclnUpwdDnwdStgDone/1 -> Logical Operator6/4
  R3RtStBkReclnUpwdDnwdStgDone/1 -> Logical Operator6/8
  [Stage1MvDone] -> EZECtrlFlow/1(Stg1done)
  [AllDone] -> AND/1
  32BitSelector/1(y) -> AND/2
  EZECtrlFlow/1(Step1En_Clear()) -> Step1En_Clear/1
  EZECtrlFlow/2(Step1En_Set()) -> Step1En_Set/1
  EZECtrlFlow/3(Step2En_Clear()) -> Step2En_Clear/1
  EZECtrlFlow/4(Step2En_Set()) -> Step2En_Set/1
  EZECtrlFlow/5(Step3En_Clear()) -> Step3En_Clear/1
  EZECtrlFlow/6(Step3En_Set()) -> Step3En_Set/1
  AND/1 -> Switch/2
  Switch/1 -> EZEMdDone/1
  Constant/1 -> Switch/1
  Switch1/1 -> Switch/3
  [AllDone] -> Switch1/2
  Constant1/1 -> Switch1/1
  Constant2/1 -> Switch1/3

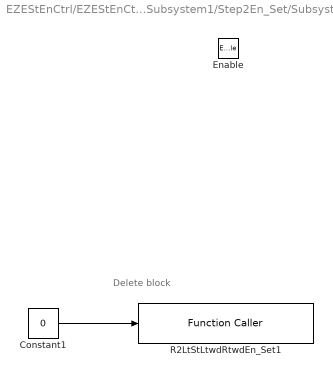
== system EZEStEnCtrl/EZEStEnCtrl_Cal_sys/Subsystem1/Step2En_Set/Subsystem ==
  note: Delete block
  Enable : EnablePort  StatesWhenEnabling=reset
  Constant1 : Constant  Value=0  OutDataTypeStr=uint8
  R2LtStLtwdRtwdEn_Set1 : FunctionCaller  FunctionPrototype=SecRwLtStLtwdRtwdEn_Set(data)  InputArgumentSpecifications=uint8(1)
  wires:
  Constant1/1 -> R2LtStLtwdRtwdEn_Set1/1

== system EZEStEnCtrl/EZEStEnCtrl_Cal_sys/Subsystem1/Step2En_Set/Subsystem1 ==
  Enable : EnablePort  StatesWhenEnabling=reset
  Constant2 : Constant  Value=0  OutDataTypeStr=uint8
  R2RtStLtwdRtwdEn_Set1 : FunctionCaller  FunctionPrototype=SecRwRtStLtwdRtwdEn_Set(data)  InputArgumentSpecifications=uint8(1)
  wires:
  Constant2/1 -> R2RtStLtwdRtwdEn_Set1/1

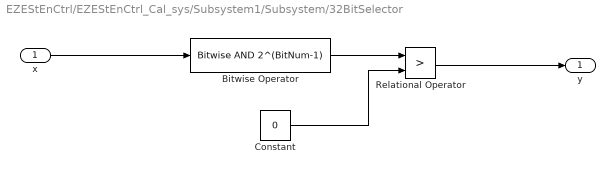
== system EZEStEnCtrl/EZEStEnCtrl_Cal_sys/Subsystem1/Subsystem/32BitSelector ==
  x : Inport
  Bitwise Operator : simulink/Logic and Bit Operations/Bitwise Operator  logicop=AND  UseBitMask=on  BitMask=2^(BitNum-1)  BitMaskRealWorld=Stored Integer
  Constant : Constant  Value=0  OutDataTypeStr=uint32
  Relational Operator : RelationalOperator  Operator=>  OutDataTypeStr=boolean  RndMeth=Simplest
  y : Outport
  wires:
  Relational Operator/1 -> y/1
  Constant/1 -> Relational Operator/2
  x/1 -> Bitwise Operator/1
  Bitwise Operator/1 -> Relational Operator/1

== stateflow chart EZEStEnCtrl/EZEStEnCtrl_Cal_sys/Subsystem1/Subsystem/EZECtrlFlow ==
  (default) -> (junction 31)
  (junction 31) -> (junction 34) [order 1] : [!Stg1done]
  (junction 31) -> (junction 38) [order 2]
  (junction 34) -> (junction 47) : {
      | Step1En_Set;
      | Step2En_Clear;
      | Step3En_Clear;
      | }
  (junction 38) -> (junction 24) [order 1] : [!Stg2done]
  (junction 38) -> (junction 43) [order 2]
  (junction 24) -> (junction 72) : {
      | Step1En_Clear;
      | Step2En_Set;
      | Step3En_Clear;
      | }
  (junction 43) -> (junction 46) [order 1] : [!Stg3done]
  (junction 43) -> (junction 71) [order 2] : {
      | Step1En_Clear;
      | Step2En_Clear;
      | Step3En_Clear;
      | }
  (junction 46) -> (junction 61) : {
      | Step1En_Clear;
      | Step2En_Clear;
      | Step3En_Set;
      | }
  (junction 61) -> (junction 71)
  (junction 72) -> (junction 61)
  (junction 47) -> (junction 72)
  (junction 71) -> (junction 48)
  data: Stg1done input boolean; Stg2done input boolean; Stg3done input boolean
  events: Step1En_Clear output FUNCTION_CALL_EVENT; Step1En_Set output FUNCTION_CALL_EVENT; Step2En_Clear output FUNCTION_CALL_EVENT; Step2En_Set output FUNCTION_CALL_EVENT; Step3En_Clear output FUNCTION_CALL_EVENT; Step3En_Set output FUNCTION_CALL_EVENT
